simulink model "DC_Motor_CoastMode_Ideal_WithGearbox"  (R2019b)
settings: Solver=VariableStepAuto  StartTime=0.0  StopTime=10.0  FixedStep=1e-5  RelTol=1e-3
InitFcn:
  | J = J_AG; % overrule motor inertia to add gearbox
settings Model: Creator=Thomas  LastModifiedBy=thomas.jespersen
settings DataIOCC: ReturnWorkspaceOutputs=off
settings DebuggingCC: ArithmeticOperatorsInVariantConditions=warning
settings SFSimCC: SimUseLocalCustomCode=off  CustomCodeUndefinedFunction=UseInterfaceOnly
settings RTWCC: RTWUseLocalCustomCode=off

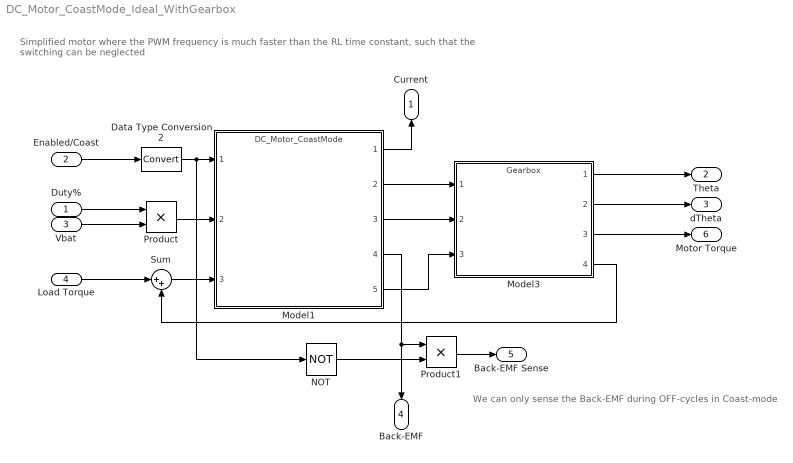
== system DC_Motor_CoastMode_Ideal_WithGearbox ==
  note: We can only sense the Back-EMF during OFF-cycles in Coast-mode
  note: Simplified motor where the PWM frequency is much faster than the RL time constant, such that the switching can be neglected
  Duty% : Inport  OutDataTypeStr=double
  Enabled/Coast : Inport  Port=2  OutDataTypeStr=boolean
  Vbat : Inport  Port=3  OutDataTypeStr=double
  Load Torque : Inport  Port=4  OutDataTypeStr=double
  Data Type Conversion2 : DataTypeConversion  RndMeth=Round
  Model1 : ModelReference  ModelNameDialog=DC_Motor_CoastMode  SimulationMode=Normal  ModelReferenceVersion=1.43
  Model3 : ModelReference  ModelNameDialog=Gearbox  SimulationMode=Normal  ModelReferenceVersion=1.7
  NOT : Logic  Operator=NOT  IconShape=distinctive  AllPortsSameDT=off  OutDataTypeStr=boolean
  Product : Product
  Product1 : Product
  Sum : Sum  Inputs=|++
  Current : Outport  VectorParamsAs1DForOutWhenUnconnected=off
  Theta : Outport  Port=2  VectorParamsAs1DForOutWhenUnconnected=off
  dTheta : Outport  Port=3  VectorParamsAs1DForOutWhenUnconnected=off
  Back-EMF : Outport  Port=4  VectorParamsAs1DForOutWhenUnconnected=off
  Back-EMF Sense : Outport  Port=5  VectorParamsAs1DForOutWhenUnconnected=off
  Motor Torque : Outport  Port=6  VectorParamsAs1DForOutWhenUnconnected=off
  wires:
  Product/1 -> Model1/2
  Enabled/Coast/1 -> Data Type Conversion2/1
  Vbat/1 -> Product/2
  Duty%/1 -> Product/1
  Model1/4 -> Back-EMF/1, Product1/1
  Data Type Conversion2/1 -> NOT/1, Model1/1
  NOT/1 -> Product1/2
  Product1/1 -> Back-EMF Sense/1
  Model1/2 -> Model3/1
  Model1/3 -> Model3/2
  Model1/5 -> Model3/3
  Model1/1 -> Current/1
  Load Torque/1 -> Sum/1
  Sum/1 -> Model1/3
  Model3/4 -> Sum/2
  Model3/1 -> Theta/1
  Model3/2 -> dTheta/1
  Model3/3 -> Motor Torque/1
